simulink model "Track_green_arduino"  (R2021b)
settings: Solver=FixedStepDiscrete  StartTime=0.0  StopTime=inf  FixedStep=0.1  RelTol=1e-3  EnableMultiTasking=on
libraries: visiontextngfix x1, dspstat3 x1, embedlinuxAVlib x1, raspberrypiCommlib x1, simulink x1, raspberrypiAVlib x1
settings Model: SimulationMode=external  ExtModeTrigDuration=100  Creator=edelaher  LastModifiedBy=litani
settings SolverCC: AlgebraicLoopSolver=TrustRegion  PositivePriorityOrder=on
settings DataIOCC: LimitDataPoints=on  SaveFormat=Array  ReturnWorkspaceOutputs=off
settings OptimizationCC: MaxStackSize=64
settings DebuggingCC: UnderspecifiedInitializationDetection=Classic  MergeDetectMultiDrivingBlocksExec=none  ParameterTunabilityLossMsg=error  AllowSymbolicDim=off  SFUnexpectedBacktrackingDiag=warning  SFNoUnconditionalDefaultTransitionDiag=warning  SFExecutionAtInitializationDiag=none  SFMachineParentedDataDiag=warning  ArithmeticOperatorsInVariantConditions=warning
settings HardwareCC: ProdBitPerPointer=32  ProdBitPerSizeT=32  ProdBitPerPtrDiffT=32  ProdLargestAtomicInteger=Long  ProdLargestAtomicFloat=Double  ProdWordSize=32  ProdHWDeviceType=ARM Compatible->ARM Cortex  UseEmbeddedCoderFeatures=off
settings ModelReferenceCC: PropagateSignalLabelsOutOfModel=off
settings SFSimCC: SimUseLocalCustomCode=off  MATLABDynamicMemAlloc=off  CustomCodeUndefinedFunction=UseInterfaceOnly
settings RTWCC: Description=Embedded Coder  SystemTargetFile=ert.tlc  HardwareBoard=Raspberry Pi  TLCOptions="-aInlineSetEventsForThisBaseRateFcn=TLC_FALSE -aSuppressMultiTaskScheduler=TLC_FALSE  -aRateBasedStepFcn=0"  TemplateMakefile=ert_default_tmf  GenerateReport=on  RTWVerbose=off  RTWUseLocalCustomCode=off  Toolchain=GNU GCC Embedded Linux  LaunchReport=on
settings CodeAppCC: ForceParamTrailComments=on  OperatorAnnotations=on  StateflowObjectComments=on  MATLABSourceComments=on
settings ERTTargetCC: MultiwordLength=2048  ERTCustomFileBanners=off  SupportContinuousTime=on  SupportNonInlinedSFcns=on  RemoveResetFunc=off  SupportVariableSizeSignals=on  ModelStepFunctionPrototypeControlCompliant=off
settings ConfigComp: CovMetricSettings=dw  CovSaveCumulativeToWorkspaceVar=on  CovSaveSingleToWorkspaceVar=on  CovExternalEMLEnable=off

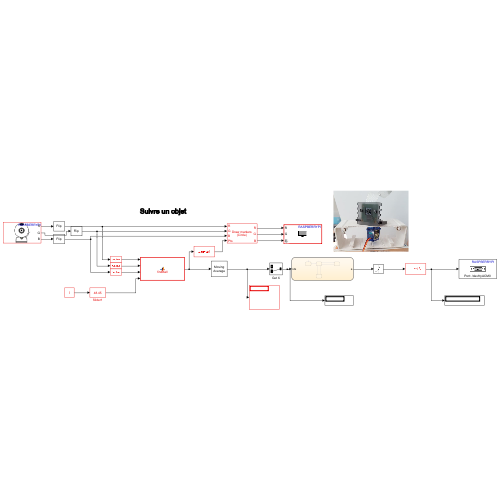
[thumbnail: Simulink's stored preview of the top-level diagram]
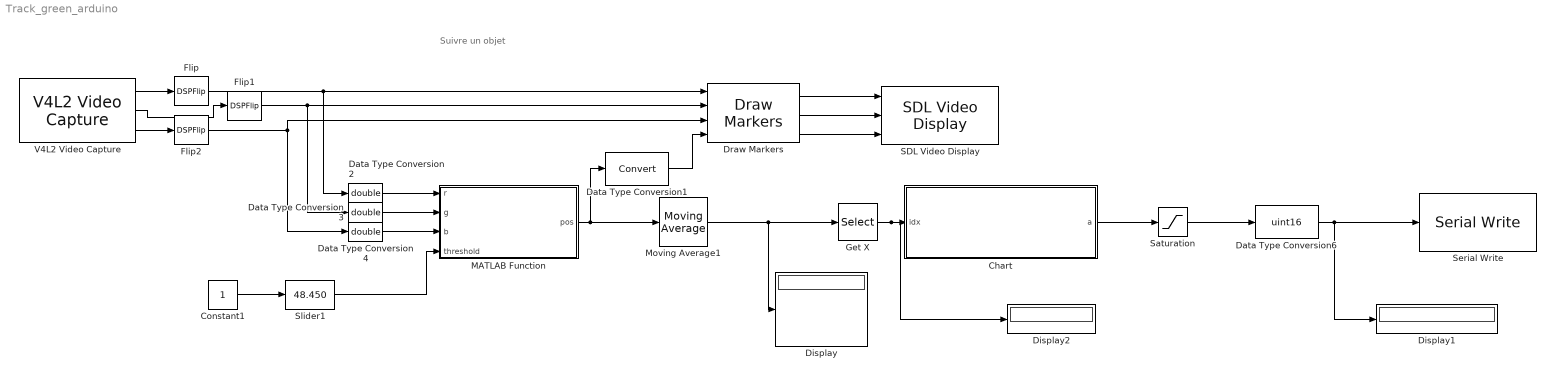
== system Track_green_arduino ==
  note: Suivre un objet
  Chart : Stateflow chart  TreatAsAtomicUnit=on
  Constant1 : Constant  OutDataTypeStr=uint8  SampleTime=0.1
  Data Type Conversion1 : DataTypeConversion
  Data Type Conversion2 : DataTypeConversion  OutDataTypeStr=double
  Data Type Conversion3 : DataTypeConversion  OutDataTypeStr=double
  Data Type Conversion4 : DataTypeConversion  OutDataTypeStr=double
  Data Type Conversion6 : DataTypeConversion  OutDataTypeStr=uint16
  Display : Display
  Display1 : Display
  Display2 : Display
  Draw Markers : visiontextngfix/Draw Markers  shape=Circle  size=3  fill=on  fillClrSource=Specify via dialog  display=User-specified value  intensity=200  color=[255 0 0]  opacity=1  viewport=Entire image  antialiasing=off  inType=Obsolete  imagePorts=Separate color signals  roundingMode=Floor  overflowMode=off  memoryMode=Specify word length  memoryWordLength=16  memoryFracLength=14  prodOutputMode=Binary point scaling  prodOutputWordLength=32  prodOutputFracLength=14
      settings: SourceProductBaseCode=VP
  Flip : DSPFlip  dim=Rows
  Flip1 : DSPFlip  dim=Rows
  Flip2 : DSPFlip  dim=Rows
  Get X : Selector  InputPortWidth=2  IndexOptions=Index vector (dialog)  Indices=2  OutputSizes=1
  MATLAB Function : MATLAB Function  TreatAsAtomicUnit=on
  Moving Average1 : dspstat3/Moving Average  Method=Sliding window  ForgettingFactorPort=off  SpecifyWindowLength=on  WindowLength=10  ForgettingFactor=0.9  SimulateUsing=Code generation
  SDL Video Display : embedlinuxAVlib/SDL Video Display  title=SDL Video Display  pixelFormat=RGB  pixelOrder=Planar  rowMajor=on  blockPlatform=Raspberry Pi
      settings: SourceProductBaseCode=SC_BEAGLEBONE_BLUE,EMBEDDEDLINUX,NVIDIA,RASPPIIO
  Saturation : Saturate  UpperLimit=110  LowerLimit=70
  Serial Write : raspberrypiCommlib/Serial Write  board=Pi 3 Model B+  SCIModule_=/dev/ttyACM0  Baudrate_=57600  Parity=None  StopBits_=1  HardwareFlowControl=None  ByteOrder=LittleEndian  OutputStatus=off  blockPlatform=RaspberryPi
      settings: SourceProductBaseCode=RASPPI
  Slider1 : simulink/Math Operations/Slider Gain  gain=48.450  low=0  high=255
  V4L2 Video Capture : raspberrypiAVlib/V4L2 Video Capture  DeviceName=/dev/video0  Resolution=320x240  CustomResolution=[ 320, 240 ]  PixelFormat=RGB  SampleTime=1/10  pixelOrder=Planar  simOutput=Colorbars  imSizeSelection=640x480  imSize=[640, 480]  roi=[0, 0, 640, 480]  m_devName='/dev/video0'  blockPlatform=Raspberry Pi
      settings: SourceProductBaseCode=RASPPI
  wires:
  V4L2 Video Capture/1 -> Flip/1
  V4L2 Video Capture/2 -> Flip1/1
  V4L2 Video Capture/3 -> Flip2/1
  Draw Markers/1 -> SDL Video Display/1
  Data Type Conversion1/1 -> Draw Markers/4
  Draw Markers/2 -> SDL Video Display/2
  Draw Markers/3 -> SDL Video Display/3
  Data Type Conversion2/1 -> MATLAB Function/1(r)
  Data Type Conversion3/1 -> MATLAB Function/2(g)
  Data Type Conversion4/1 -> MATLAB Function/3(b)
  Slider1/1 -> MATLAB Function/4(threshold)
  Constant1/1 -> Slider1/1
  Moving Average1/1 -> Display/1, Get X/1
  Get X/1 -> Display2/1, Chart/1(idx)
  MATLAB Function/1(pos) -> Moving Average1/1, Data Type Conversion1/1
  Data Type Conversion6/1 -> Display1/1, Serial Write/1
  Chart/1(a) -> Saturation/1
  Saturation/1 -> Data Type Conversion6/1
  Flip/1 -> Draw Markers/1, Data Type Conversion2/1
  Flip1/1 -> Data Type Conversion3/1, Draw Markers/2
  Flip2/1 -> Data Type Conversion4/1, Draw Markers/3

== matlab function Track_green_arduino/MATLAB Function ==
  data: r input; g input; b input; pos output; threshold input
function pos = findBall(r,g,b,threshold)
%#codegen
%% Calculate Green
% Then we perform an arithmetic operation on the matrices as a whole to try
% to create one matrix that represents an intensity of green.
justGreen = g - r/2 - b/2;

%% Threshold the image
% Now we can set a threshold to separate the parts of the image that we
% consider to be green from the rest.
bw = justGreen > threshold;

%% Find center
% Find the row and column location of the pixels and calculate the mean to get
% the approximate center of the ball.
[r,c] = find(bw);
if isempty(r)
    pos = [0 0];
else
    pos = [mean(c) mean(r)];
end

== stateflow chart Track_green_arduino/Chart ==
  state Init
    en: a=90;
  state rien
    %onf fait rien
  state gauche
    a=a-1;
  state droite
    a=a+1;
  (default) -> Init
  rien -> gauche [order 2] : [idx-320<-20]
  Init -> rien
  gauche -> rien : [abs(idx-320)<20]
  rien -> droite [order 1] : [idx-320>20]
  droite -> rien : [abs(idx-320)<20]
  data: idx input; a output
